simulink model "Lithium0x2Dion"  (R2024b)
settings: Solver=FixedStepAuto  StartTime=0.0  StopTime=1000  FixedStep=0.001  RelTol=1e-3
libraries: spsControlledCurrentSourceLib x1, spsControlledVoltageSourceLib x1, spsCurrentMeasurementLib x1, spsSeriesRLCBranchLib x1, spsVoltageMeasurementLib x1, sps_lib x1
(part 1 of 3)
settings Model: Creator=holthoff  LastModifiedBy=kauchr

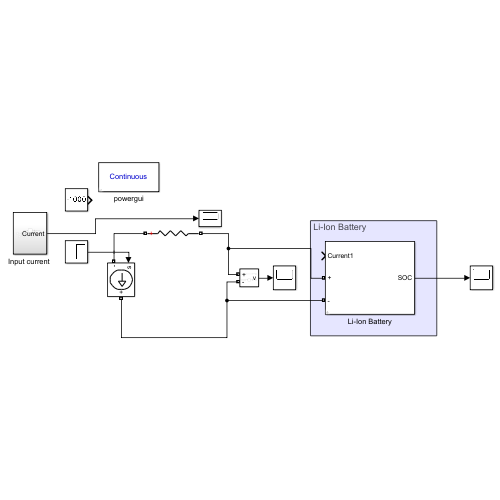
[thumbnail: Simulink's stored preview of the top-level diagram]
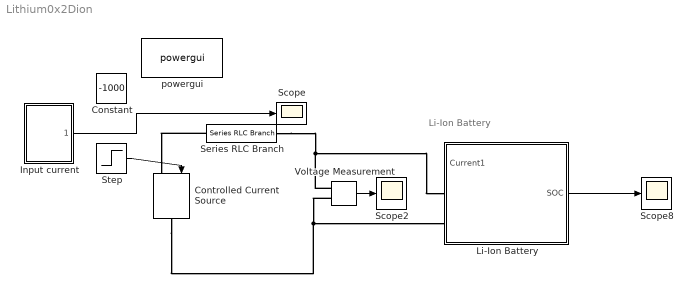
== system Lithium0x2Dion ==
  note: Li-Ion Battery
  Constant : Constant  Value=-1000
  Controlled Current Source : spsControlledCurrentSourceLib/Controlled Current Source  Initialize=off  Source_Type=AC  Amplitude=0  Phase=0  Frequency=0  Measurements=None
  "Input current " : Subsystem
  Li-Ion Battery : Subsystem  mask{RCap=1000, NomV=500, soc=50, Battime=10}
      mask prompts: RCap "Rated Capacity (Ah)"; NomV "Nominal Voltage (V)"; soc "Initial SOC (%)"; Battime "Battery Response Time (s)"
  Scope : Scope
  Scope2 : Scope
  Scope8 : Scope
  Series RLC Branch : spsSeriesRLCBranchLib/Series RLC Branch  LConnTagsString=__new0  RConnTagsString=__new0  BranchType=R  Resistance=1  Inductance=1e-3  SetiL0=off  InitialCurrent=0  Capacitance=1e-6  Setx0=off  InitialVoltage=0  Measurements=None
  Step : Step  Time=100  After=100  SampleTime=0
  Voltage Measurement : spsVoltageMeasurementLib/Voltage Measurement  PhasorSimulation=off  OutputType=Complex  PSBequivalent=0
  powergui : sps_lib/powergui  Priority=1  SimulationMode=Continuous  SampleTime=50e-6  frequency=60  Iterations=50  frequencyindice=0  Pbase=100e6  ErrMax=1e-4  UnitsV=kV  UnitsW=MW  buscounter=0  FunctionMessages=off  echomessages=off  EnableUseOfTLC=off  CurrentSourceSwitches=off  DisableSnubberDevices=off  DisableRonSwitches=off  DisableVfSwitches=off  DisplayEquations=off  AutomaticDiscreteSolvers=off  SolverType=Tustin/Backward Euler (TBE)  Interpol=off  ExternalGateDelay=off  methode=off  Ts=100  x0status=blocks  SPID=on  SwTol=0  HookPort=off  NonlinearTolerance=1e-4  nMaxIteration=100  ContinueOnMaxIteration=off  RestoreLinks=warning  ResistiveCurrentMeasurement=off  Frange=[0:2:500]  Ylog=off  Xlog=on  ShowGrid=off  save=off  variable=ZData  structure=0  ZoomFFT=off  StartTime=0.0  cycles=1  DisplayStyle=1  fundamental=60  FreqAxis=off  MaxFrequency=1000  frequencyindicesteady=1  RmsSteady=1  display=off
  wires:
  "Input current "/1(Current) -> Scope/1
  Li-Ion Battery/1(SOC) -> Scope8/1
  Voltage Measurement/1 -> Scope2/1
  Step/1 -> Controlled Current Source/1
  connections:
  Controlled Current Source/RConn1 -- Voltage Measurement/LConn2 -- Li-Ion Battery/LConn2
  Voltage Measurement/LConn1 -- Series RLC Branch/RConn1 -- Li-Ion Battery/LConn1
  Series RLC Branch/LConn1 -- Controlled Current Source/LConn1
